simulink model "cycleABC1"  (Simulink 8.5)
settings: Solver=ode1  StartTime=0.0  StopTime=Inf  FixedStep=0.005  RelTol=1e-3
libraries: simulink x5
settings Model: Creator=bbarbedette  LastModifiedBy=ryad.boukhari
settings OptimizationCC: BlockReduction=off  OptimizeBlockIOStorage=off  BufferReuse=off  GlobalBufferReuse=off  ExpressionFolding=off  LocalBlockOutputs=off  InitFltsAndDblsToZero=on
settings DebuggingCC: SaveWithParameterizedLinksMsg=none  SolverPrmCheckMsg=warning  FcnCallInpInsideContextMsg=UseLocalSettings
settings HardwareCC: ProdIntDivRoundTo=Zero  ProdEndianess=BigEndian  ProdHWDeviceType=Specified  TargetIntDivRoundTo=Zero  TargetEndianess=BigEndian
settings RTWCC: SystemTargetFile=rti1401.tlc  MakeCommand=make_rti  TemplateMakefile=rti1401.tmf  Description=dSPACE DS1401 Hardware Platform
settings STFCustomTargetCC: TargetFcnLib=ansi_tfl_tmw.mat  ModelReferenceCompliant=off  GeneratePreprocessorConditionals=Disable all  MatFileLogging=on  CPPClassGenCompliant=on  SystemTargetFile=rti1401.tlc
settings GRTTargetCC: TargetFcnLib=ansi_tfl_tmw.mat  ModelReferenceCompliant=off  ParMdlRefBuildCompliant=off  CompOptLevelCompliant=off  ConcurrentExecutionCompliant=off  ExtModeMexFile=noextcomm
settings CustomProperty: DataType=RTWOptions_EnumType_c__dspace_matlab_rti1401_tlc_rti1401_InitialSimState  Value=RUN
settings EnumStrPairs: String=RUN

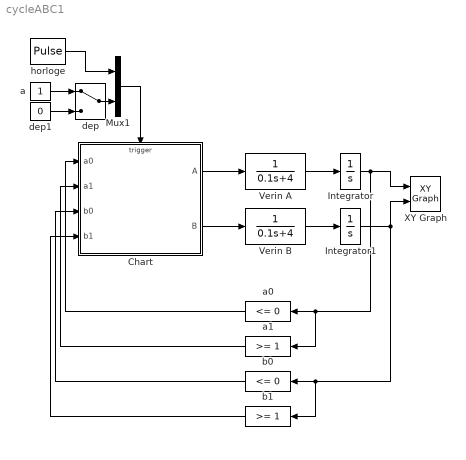
== system cycleABC1 ==
  Chart : Stateflow chart  TreatAsAtomicUnit=on
  Integrator : Integrator
  Integrator1 : Integrator
  Mux1 : Mux  Inputs=2
  Verin A : TransferFcn  Denominator=[0.1 4]
  Verin B : TransferFcn  Denominator=[0.1 4]
  XY Graph : simulink/Sinks/XY Graph  xmin=-3  xmax=3  ymin=-3  ymax=3  st=-1
  a : Constant
  a0 : simulink/Logic and Bit Operations/Compare To Constant  relop=<=  const=0  OutDataTypeStr=uint8  ZeroCross=off
  a1 : simulink/Logic and Bit Operations/Compare To Constant  relop=>=  const=1  OutDataTypeStr=uint8  ZeroCross=off
  b0 : simulink/Logic and Bit Operations/Compare To Constant  relop=<=  const=0  OutDataTypeStr=uint8  ZeroCross=off
  b1 : simulink/Logic and Bit Operations/Compare To Constant  relop=>=  const=1  OutDataTypeStr=uint8  ZeroCross=off
  dep : ManualSwitch
  dep1 : Constant  Value=0
  horloge : DiscretePulseGenerator  PulseType=Time based  Period=.01  PulseWidth=50
  wires:
  a/1 -> dep/1
  horloge/1 -> Mux1/1
  dep/1 -> Mux1/2
  Mux1/1 -> Chart/Trigger
  dep1/1 -> dep/2
  Chart/1(A) -> Verin A/1
  Chart/2(B) -> Verin B/1
  Verin A/1 -> Integrator/1
  Verin B/1 -> Integrator1/1
  a0/1 -> Chart/1(a0)
  a1/1 -> Chart/2(a1)
  b0/1 -> Chart/3(b0)
  b1/1 -> Chart/4(b1)
  Integrator/1 -> XY Graph/1, a0/1, a1/1
  Integrator1/1 -> XY Graph/2, b0/1, b1/1

== stateflow chart Chart ==
  state X0
    en:A=0;B=0
  state X1
    en:A=1
  state X2
    en:A=0;B=1;
  state X3
    en:
    B=0;A=-1;
    B=-1
  (default) -> X0
  X3 -> X0 : [a0==1&b0==1]
  X0 -> X1 : dep[a0==1&b0==1]
  X1 -> X2 : [a1==1]
  X2 -> X3 : [b1==1]
  data: a0 input double; a1 input double; b0 input double; b1 input double; A output double; B output double
  events: horloge input RISING_EDGE_EVENT; dep input RISING_EDGE_EVENT
